simulink model "Simulation_1_3_dof"  (R2025a)
settings: Solver=VariableStepAuto  StartTime=0.0  StopTime=2000  FixedStep=1e-3  RelTol=1e-3
model workspace (MAT data in the model file):
  L1 = 0.29412
  L2 = 0.366795
  data_in = [0 0 0.1183997 0.1183997 0.1183997 0.03355169 0.03355169 0.3118325 0.3118325 0.3118325 0.3118325 0.6475105 ... (368 elements, 1x368)]
  data_in2 = [0 0 0 -1.210024 -1.210024 -1.210024 -1.304783 -1.304783 -1.304783 -1.673209 -1.673209 -1.673209 ... (368 elements, 1x368)]
  data_inYZ = [3.321716 3.321716 2.118667 2.118667 2.118667 2.649823 2.649823 2.756135 2.756135 2.756135 2.756135 2.832357 ... (368 elements, 1x368)]
  g = 9.81
  m1 = 1.7875
  m2 = 1.0285
  m3 = 0.3575
  m3_new = 2.3575
  m3_state_input = [0 0 0 0 0 0 0 0 0 0 0 0 0 0 0 0 0 0 0 0 0 0 0 0 0 0 0 0 0 0 0 0 0 0 0 0 0 0 0 0 0 0 0 0 0 0 0 0 0 0 0 0 0 0 0 0 0 0 0 0 0 0 0 0 0 0 0 0 0 0 0 0 0 0 0 0 0 0 0 0 0 0 0 0 0 0 0 0 0 0 0 0 0 0 0 0 0 0 0 0 0 0 0 0 0 0 0 0 0 0 0 0 0 0 0 0 0 0 0 0 0 0 0 0 0 0 0 0 0 0 0 0 0 0 0 0 0 0 0 0 0 0 0 0 0 0 0 0 0 0 0 0 0 0 0 0 0 0 0 0 0 0 0 0 0 0 0 0 0 0 0 0 0 0 0 0 0 0 0 0 0 0 0 0 0 0 0 0 0 0 0 0 0 0 0 0 0 0 0 0 0 0 0 0 0 0 0 0 0 0 0 0 0 0 0 0 0 0 0 0 0 0 0 0 0 0 0 0 0 0 0 0 0 0 0 0 0 0 0 0 0 0 0 0 0 0 0 0 0 0 0 0 0 0 0 0 0 0 0 0 0 0 0 0 0 0 0 0 0 0 0 0 0 0 0 0 0 0 0 0 0 0 0 0 0 0 0 0 0 0 0 0 0 0 0 0 0 0 0 0 0 0 0 0 0 0 0 0 0 0 0 0 0 0 0 0 0 0 0 0 0 0 0 0 0 0 0 0 0 0 0 0 0 0 0 0 0 0 0 0 0 0 0 0 0 0 0 0 0 0 0 0 0 0 0 0 0 0 0 0 0 0 0 0 0 0 0 0]
  trial_length = 12.6
libraries: simulink x1, slctrl_adaptive x1
settings Model: Creator=Queen  LastModifiedBy=jaanr
settings SolverCC: MaxConsecutiveMinStep=20  ZeroCrossAlgorithm=Adaptive
settings DataIOCC: SaveState=on
settings DebuggingCC: SignalInfNanChecking=warning  AlgebraicLoopMsg=none  IgnoredZcDiagnostic=none  SolverPrmCheckMsg=warning  CheckMatrixSingularityMsg=warning  StateNameClashWarn=warning  UnderSpecifiedDimensionMsg=warning

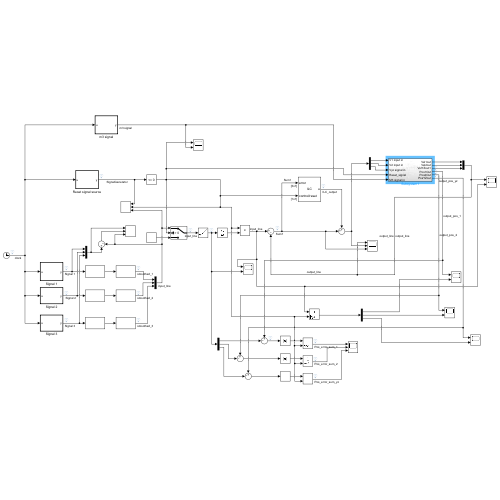
[thumbnail: Simulink's stored preview of the top-level diagram]
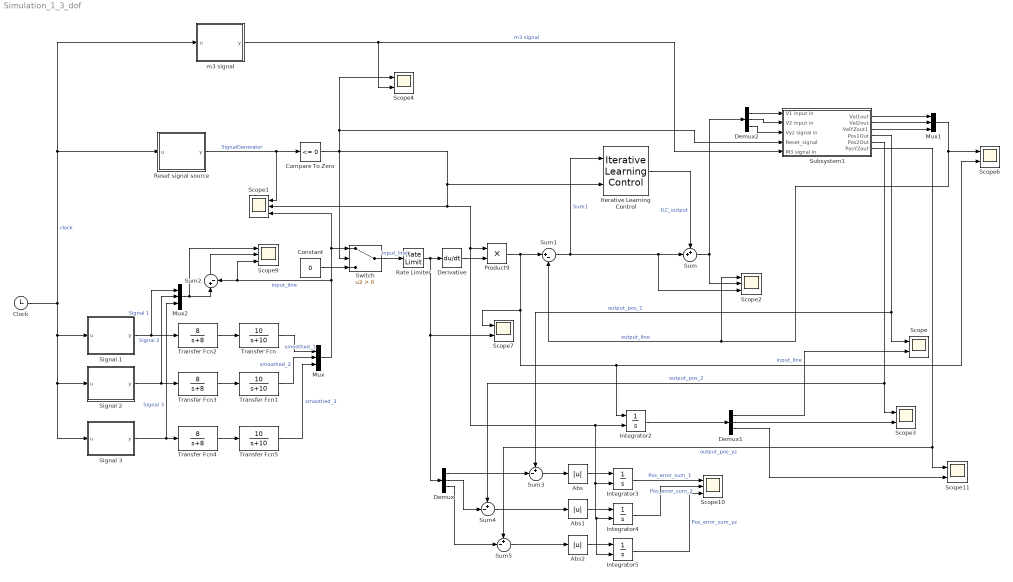
== system Simulation_1_3_dof ==
  Abs : Abs  SaturateOnIntegerOverflow=off
  Abs1 : Abs  SaturateOnIntegerOverflow=off
  Abs2 : Abs  SaturateOnIntegerOverflow=off
  Clock : Clock
  Compare To Zero : simulink/Logic and Bit Operations/Compare To Zero  relop=<=  OutDataTypeStr=boolean
  Constant : Constant  Value=0
  Demux : Demux  Outputs=3
  Demux1 : Demux  Outputs=3
  Demux2 : Demux  Outputs=3
  Derivative : Derivative
  Integrator{2..5} (4 alike) : Integrator  ExternalReset=either
  Iterative Learning Control : slctrl_adaptive/Iterative Learning Control  Ts=0.004  Tspan=trial_length  dataType=double  Algorithm=Model based ILC  gamma_p=1  gamma_d=0  ModelTimeDomain=Continuous time  A=[0 0 0; 0 0 0; 0 0 0]  B=[1 0 0; 0 1 0; 0 0 1]  C=[1 0 0; 0 1 0; 0 0 1]  ModelBasedILCType=Inverse-model based  gamma_inverse=1.9  gamma_grad=1  LPFEnable=on  tau=10
      settings: LibrarySourceBlock=slctrlblks/Adaptive Control/Iterative Learning Control
  Mux : Mux  Inputs=3
  Mux1 : Mux  Inputs=3
  Mux2 : Mux  Inputs=3
  Product9 : Product
  Rate Limiter : RateLimiter  RisingSlewLimit=100000  FallingSlewLimit=-100000  SampleTimeMode=inherited
  Reset signal source : MATLAB Function  StartFcn=const = data_in;  TreatAsAtomicUnit=on
  Scope{,3..4,6..7,11} (6 alike) : Scope  NumInputPorts=2
      Scope settings: ActiveDisplayYMinimum=-13.826115820369353  ActiveDisplayYMaximum=226.98217036515493
      Scope11 settings: ActiveDisplayYMinimum=-0.18701704840304334  ActiveDisplayYMaximum=1.1318992906932446  DataLoggingVariableName=ScopeData8
      Scope3 settings: ActiveDisplayYMinimum=-8.2804975413162367  ActiveDisplayYMaximum=200.54991353193529  DataLoggingVariableName=ScopeData3
      Scope4 settings: ActiveDisplayYMinimum=0.10884484415759765  ActiveDisplayYMaximum=4.3831313228801481
      Scope6 settings: ActiveDisplayYMinimum=-322.72558200957525  ActiveDisplayYMaximum=537.26898968089313  DataLoggingVariableName=ScopeData2
      Scope7 settings: ActiveDisplayYMinimum=-257.38444532138942  ActiveDisplayYMaximum=191.12119574725739  DataLoggingVariableName=ScopeData4
  Scope{1..2,9..10} (4 alike) : Scope  NumInputPorts=3
      Scope1 settings: ActiveDisplayYMinimum=80.127820191653512  ActiveDisplayYMaximum=87.873782524375827
      Scope10 settings: ActiveDisplayYMinimum=-1  ActiveDisplayYMaximum=1  DataLoggingVariableName=ScopeData7
      Scope2 settings: ActiveDisplayYMinimum=13.345255866197224  ActiveDisplayYMaximum=15.321548211532381  DataLoggingVariableName=ScopeData2
      Scope9 settings: ActiveDisplayYMinimum=-59.300205634382507  ActiveDisplayYMaximum=210.11663457106687  DataLoggingVariableName=ScopeData5
  Signal 1 : MATLAB Function  StartFcn=const = data_in;  TreatAsAtomicUnit=on
  Signal 2 : MATLAB Function  TreatAsAtomicUnit=on
  Signal 3 : MATLAB Function  TreatAsAtomicUnit=on
  Subsystem1 : Subsystem
  Sum : Sum  Inputs=++|
  Sum1 : Sum  Inputs=|+-
  Sum2 : Sum  Inputs=|+-
  Sum3 : Sum  Inputs=+-|
  Sum4 : Sum  Inputs=+-|
  Sum5 : Sum  Inputs=+-|
  Switch : Switch  Criteria=u2 > Threshold  SaturateOnIntegerOverflow=off  InputSameDT=off
  Transfer Fcn : TransferFcn  Numerator=[10]  Denominator=[1 10]
  Transfer Fcn1 : TransferFcn  Numerator=[10]  Denominator=[1 10]
  Transfer Fcn2 : TransferFcn  Numerator=[8]  Denominator=[1 8]
  Transfer Fcn3 : TransferFcn  Numerator=[8]  Denominator=[1 8]
  Transfer Fcn4 : TransferFcn  Numerator=[8]  Denominator=[1 8]
  Transfer Fcn5 : TransferFcn  Numerator=[10]  Denominator=[1 10]
  m3 signal : MATLAB Function  StartFcn=const = data_in;  TreatAsAtomicUnit=on
  wires:
  Constant/1 -> Switch/3
  Reset signal source/1(y) -> Scope1/1, Compare To Zero/1  "SignalGenerator"
  Compare To Zero/1 -> Integrator5/2, Integrator4/2, Integrator3/2, Integrator2/2, Product9/1, Scope1/2, Iterative Learning Control/2, Subsystem1/4(Reset_signal), Scope4/1, Switch/2
  Product9/1 -> Integrator2/1, Scope6/2, Scope7/1, Sum1/1  "input_line"
  Sum1/1 -> Sum/2, Scope2/3, Iterative Learning Control/1  "Sum1"
  Sum/1 -> Scope2/2, Demux2/1
  Mux1/1 -> Sum1/2, Scope2/1, Scope6/1  "output_line"
  Clock/1 -> m3 signal/1(u), Reset signal source/1(u), Signal 3/1(u), Signal 2/1(u), Signal 1/1(u)  "clock"
  Subsystem1/4(Pos1Out) -> Scope/1, Sum3/1  "output_pos_1"
  Subsystem1/5(Pos2Out) -> Sum4/1, Scope3/1  "output_pos_2"
  Demux1/1 -> Scope/2
  Demux1/2 -> Scope3/2
  Signal 2/1(y) -> Transfer Fcn3/1, Mux2/2  "Signal 2"
  Subsystem1/1(Vel1out) -> Mux1/1
  Subsystem1/2(Vel2out) -> Mux1/2
  Demux2/1 -> Subsystem1/1(V1 input in)
  Demux2/2 -> Subsystem1/2(V2 input in)
  Iterative Learning Control/1 -> Sum/1  "ILC_output"
  Integrator2/1 -> Demux1/1
  Switch/1 -> Rate Limiter/1  "input_line"
  Derivative/1 -> Product9/2
  Rate Limiter/1 -> Derivative/1, Demux/1, Scope7/2
  Signal 1/1(y) -> Transfer Fcn2/1, Mux2/1  "Signal 1"
  Mux/1 -> Scope9/3, Sum2/2, Scope1/3, Switch/1  "input_line"
  Transfer Fcn/1 -> Mux/1  "smoothed_1"
  Transfer Fcn1/1 -> Mux/2  "smoothed_2"
  Mux2/1 -> Sum2/1, Scope9/1
  Sum2/1 -> Scope9/2
  Transfer Fcn2/1 -> Transfer Fcn/1
  Transfer Fcn3/1 -> Transfer Fcn1/1
  m3 signal/1(y) -> Scope4/2, Subsystem1/5(M3 signal in)  "m3 signal"
  Demux/1 -> Sum3/2
  Demux/2 -> Sum4/2
  Sum3/1 -> Abs/1
  Sum4/1 -> Abs1/1
  Integrator3/1 -> Scope10/1  "Pos_error_sum_1"
  Integrator4/1 -> Scope10/2  "Pos_error_sum_2"
  Abs/1 -> Integrator3/1
  Abs1/1 -> Integrator4/1
  Signal 3/1(y) -> Transfer Fcn4/1, Mux2/3  "Signal 3"
  Transfer Fcn4/1 -> Transfer Fcn5/1
  Transfer Fcn5/1 -> Mux/3  "smoothed_3"
  Demux/3 -> Sum5/2
  Subsystem1/3(VelYZout1) -> Mux1/3
  Demux1/3 -> Scope11/2
  Subsystem1/6(PosYZout) -> Sum5/1, Scope11/1  "output_pos_yz"
  Sum5/1 -> Abs2/1
  Abs2/1 -> Integrator5/1
  Integrator5/1 -> Scope10/3  "Pos_error_sum_yz"
  Demux2/3 -> Subsystem1/3(Vyz signal in)

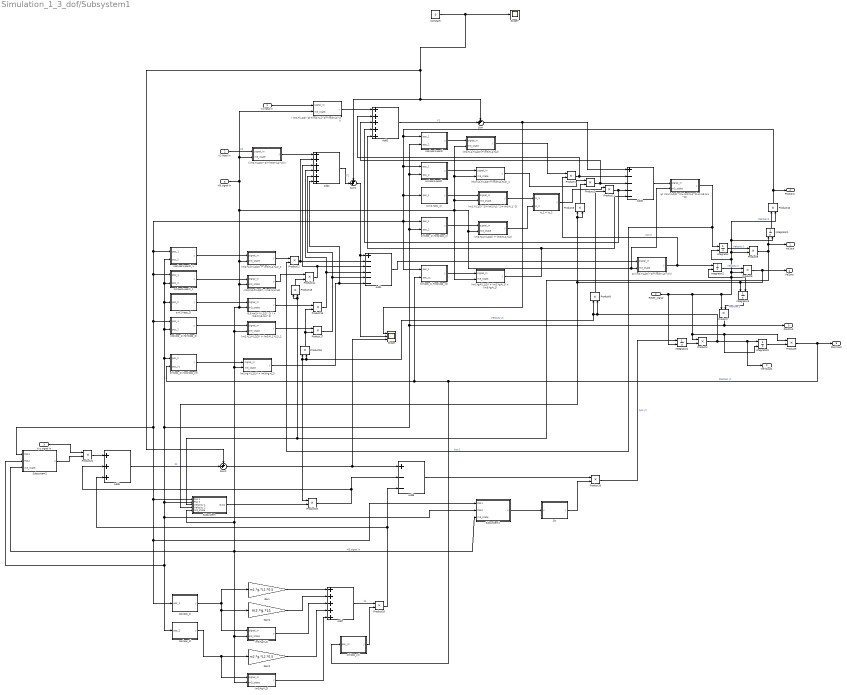
== system Simulation_1_3_dof/Subsystem1 ==
  V1 input in : Inport
  V2 input in : Inport  Port=2
  Vyz signal in : Inport  Port=3
  Reset_signal : Inport  Port=4
  M3 signal in : Inport  Port=5
  ( (m1.*(L1/2)^2)+(m2.*L1^2)+(m3.*L1^2)) : MATLAB Function  TreatAsAtomicUnit=on
  ((m2.*(L2/2)^2)+(m3.*(L2^2))) : MATLAB Function  TreatAsAtomicUnit=on
  (0.5.*m2.* ((L2/2)^2) ) + (0.5.*m3.*L2^2) : MATLAB Function  TreatAsAtomicUnit=on
  (m1.*(L1/2)^2)+(m2.*L1^2)+(m3.*L1^2) : MATLAB Function  TreatAsAtomicUnit=on
  (m1.*g.*(L1/2)) + (m2.*g.*L1) + (m3.*g.*L1) : MATLAB Function  TreatAsAtomicUnit=on
  (m2.*L1.*(L2/2)) + (m3.*L1.*L2) : MATLAB Function  TreatAsAtomicUnit=on
  (m2.*L1.*(L2/2)) + (m3.*L1.*L2)_1 : MATLAB Function  TreatAsAtomicUnit=on
  (m2.*L1.*(L2/2)) + (m3.*L1.*L2)_2 : MATLAB Function  TreatAsAtomicUnit=on
  (m2.*L1.*(L2/2))+(m3.*L1.*L2) : MATLAB Function  TreatAsAtomicUnit=on
  (m2.*L1.*(L2/2))+(m3.*L1.*L2)_1 : MATLAB Function  TreatAsAtomicUnit=on
  (m2.*g.*(L2/2)) + (m3.*g.*L2) : MATLAB Function  TreatAsAtomicUnit=on
  (m3.*g.*L1) : MATLAB Function  TreatAsAtomicUnit=on
  (m3.*g.*L2) : MATLAB Function  TreatAsAtomicUnit=on
  -(m2.*L1.*(L2/2)) - (m3.*L1.*L2) : MATLAB Function  TreatAsAtomicUnit=on
  1/( (m1.*(L1/2)^2)+(m2.*L1^2)+(m3.*L1^2)) : MATLAB Function  TreatAsAtomicUnit=on
  1/( (m2.*(L2/2)^2)+(m3.*(L2^2))) : MATLAB Function  TreatAsAtomicUnit=on
  1/u : MATLAB Function  TreatAsAtomicUnit=on
  Add1 : Sum  Inputs=+-----
  Add2 : Sum  Inputs=+++++
  Add3 : Sum  Inputs=+----
  Add4 : Sum  Inputs=++++++
  Add5 : Sum  Inputs=+++
  Add6 : Sum  Inputs=+--
  Add7 : Sum  Inputs=+++++
  Constant : Constant  Value=0
  Gain : Gain  Gain=m1.*g.*L1.*0.5
  Gain1 : Gain  Gain=m2.*g.*L1
  Gain2 : Gain  Gain=m2.*g.*L2.*0.5
  Integrator{,1..5} (6 alike) : Integrator  ExternalReset=either
  Product{1..21} (21 alike) : Product
  Scope : Scope  NumInputPorts=3
      settings: DataLoggingVariableName=ScopeData9
  Scope7 : Scope
      settings: ActiveDisplayYMinimum=-1  ActiveDisplayYMaximum=1  DataLoggingVariableName=ScopeData6
  Subsystem : Subsystem
  Subsystem1 : Subsystem
  Subsystem2 : Subsystem
  Sum : Sum  Inputs=++|
  Sum1 : Sum  Inputs=++|
  Sum2 : Sum  Inputs=++|
  cos(pos1-pos2) : MATLAB Function  TreatAsAtomicUnit=on
  cos(pos1-pos2)_1 : MATLAB Function  TreatAsAtomicUnit=on
  cos(pos_1) : MATLAB Function  TreatAsAtomicUnit=on
  cos(pos_1).*sin(pos_2) : MATLAB Function  TreatAsAtomicUnit=on
  cos(pos_2) : MATLAB Function  TreatAsAtomicUnit=on
  in_1 + in_2 : MATLAB Function  TreatAsAtomicUnit=on
  sin(2.*pos_1) : MATLAB Function  TreatAsAtomicUnit=on
  sin(2.*pos_2) : MATLAB Function  TreatAsAtomicUnit=on
  sin(pos1-pos2) : MATLAB Function  TreatAsAtomicUnit=on
  sin(pos1-pos2)_1 : MATLAB Function  TreatAsAtomicUnit=on
  sin(pos_1).*cos(pos_2) : MATLAB Function  TreatAsAtomicUnit=on
  sin(pos_1).*cos(pos_yz) : MATLAB Function  TreatAsAtomicUnit=on
  sin(pos_2).*cos(pos_yz) : MATLAB Function  TreatAsAtomicUnit=on
  sin(pos_yz) : MATLAB Function  TreatAsAtomicUnit=on
  Vel1out : Outport
  Vel2out : Outport  Port=2
  VelYZout1 : Outport  Port=3
  Pos1Out : Outport  Port=4
  Pos2Out : Outport  Port=5
  PosYZout : Outport  Port=6
  wires:
  Product9/1 -> Vel1out/1, Integrator1/1, Subsystem/3(Velocity 1), Product13/2, Product13/1
  Product6/1 -> Vel2out/1, Subsystem/4(Velocity 2), Product3/2, Product3/1, Integrator3/1
  Add3/1 -> 1/( (m1.*(L1/2)^2)+(m2.*L1^2)+(m3.*L1^2))/1(signal_in)
  1/( (m1.*(L1/2)^2)+(m2.*L1^2)+(m3.*L1^2))/1(y) -> Product12/2, Integrator/1  "Acc 1"
  Product10/1 -> cos(pos1-pos2)/1(pos_1), sin(pos1-pos2)/1(pos_1), sin(pos_1).*cos(pos_yz)/1(pos_1), cos(pos_1).*sin(pos_2)/1(pos_1), Subsystem1/1(Pos1), cos(pos_1)/1(pos_1), Subsystem/1(Pos 1), Subsystem2/1(Pos1), sin(pos1-pos2)_1/1(pos_1), cos(pos1-pos2)_1/1(pos_1), sin(pos_1).*cos(pos_2)/1(pos_1), sin(2.*pos_1)/1(pos_1), Pos1Out/1
  Product7/1 -> cos(pos_1).*sin(pos_2)/2(pos_2), sin(2.*pos_2)/1(pos_2), sin(pos1-pos2)_1/2(pos_2), cos(pos1-pos2)_1/2(pos_2), sin(pos_2).*cos(pos_yz)/1(pos_2), Subsystem2/2(Pos2), cos(pos_2)/1(pos_2), Subsystem1/2(Pos2), Subsystem/2(Pos 2), sin(pos1-pos2)/2(pos_2), cos(pos1-pos2)/2(pos_2), sin(pos_1).*cos(pos_2)/2(pos_2), Pos2Out/1
  1/( (m2.*(L2/2)^2)+(m3.*(L2^2)))/1(y) -> Product1/2, Integrator2/1  "Acc 2"
  Add1/1 -> 1/( (m2.*(L2/2)^2)+(m3.*(L2^2)))/1(signal_in)
  ( (m1.*(L1/2)^2)+(m2.*L1^2)+(m3.*L1^2))/1(y) -> Add2/1
  V1 input in/1 -> ( (m1.*(L1/2)^2)+(m2.*L1^2)+(m3.*L1^2))/1(signal_in)
  V2 input in/1 -> ((m2.*(L2/2)^2)+(m3.*(L2^2)))/1(signal_in)  "F2"
  ((m2.*(L2/2)^2)+(m3.*(L2^2)))/1(y) -> Add4/1
  Sum/1 -> Scope/1, Add3/1
  Constant/1 -> Sum2/1, Sum1/1, Sum/1, Scope7/1
  Sum1/1 -> Scope/2, Add1/1
  Add2/1 -> Sum/2  "F1"
  Add4/1 -> Sum1/2  "F2"
  Integrator/1 -> Product9/1  "Velocity 1"
  Integrator1/1 -> Product10/1  "Position 1"
  Integrator2/1 -> Product6/1  "Velocity 2"
  Integrator3/1 -> Product7/2  "Position 2"
  Reset_signal/1 -> Integrator4/2, Product10/2, Integrator1/2, Product9/2, Integrator/2, Product6/2, Integrator3/2, Integrator2/2, Product7/1, Product5/1, Integrator5/2, Product4/1
  M3 signal in/1 -> (m1.*g.*(L1/2)) + (m2.*g.*L1) + (m3.*g.*L1)/2(m3_state), 1/( (m1.*(L1/2)^2)+(m2.*L1^2)+(m3.*L1^2))/2(m3_state), 1/( (m2.*(L2/2)^2)+(m3.*(L2^2)))/2(m3_state), (m2.*L1.*(L2/2)) + (m3.*L1.*L2)/2(m3_state), (m1.*(L1/2)^2)+(m2.*L1^2)+(m3.*L1^2)/2(m3_state), (m2.*L1.*(L2/2))+(m3.*L1.*L2)/2(m3_state), (m2.*L1.*(L2/2))+(m3.*L1.*L2)_1/2(m3_state), -(m2.*L1.*(L2/2)) - (m3.*L1.*L2)/2(m3_state), (0.5.*m2.* ((L2/2)^2) ) + (0.5.*m3.*L2^2)/2(m3_state), (m2.*L1.*(L2/2)) + (m3.*L1.*L2)_2/2(m3_state), (m2.*g.*(L2/2)) + (m3.*g.*L2)/2(m3_state), Subsystem1/3(m3_state), (m3.*g.*L2)/2(m3_state), (m3.*g.*L1)/2(m3_state), Subsystem2/3(m3_state), Subsystem/5(m3_state), (m2.*L1.*(L2/2)) + (m3.*L1.*L2)_1/2(m3_state), ( (m1.*(L1/2)^2)+(m2.*L1^2)+(m3.*L1^2))/2(m3_state), ((m2.*(L2/2)^2)+(m3.*(L2^2)))/2(m3_state)  "M3 signal in"
  cos(pos1-pos2)/1(y) -> (m2.*L1.*(L2/2))+(m3.*L1.*L2)/1(signal_in)
  (m2.*L1.*(L2/2))+(m3.*L1.*L2)/1(y) -> Product1/1
  Product1/1 -> Add2/2, Add3/2
  sin(pos1-pos2)/1(y) -> (m2.*L1.*(L2/2))+(m3.*L1.*L2)_1/1(signal_in)
  (m2.*L1.*(L2/2))+(m3.*L1.*L2)_1/1(y) -> Product2/1
  Product3/1 -> Product2/2
  Product2/1 -> Add2/3, Add3/3
  sin(2.*pos_1)/1(y) -> (m1.*(L1/2)^2)+(m2.*L1^2)+(m3.*L1^2)/1(signal_in)
  (m1.*(L1/2)^2)+(m2.*L1^2)+(m3.*L1^2)/1(y) -> in_1 + in_2/1(in_1)
  sin(pos_1).*cos(pos_2)/1(y) -> (m2.*L1.*(L2/2)) + (m3.*L1.*L2)/1(signal_in)
  (m2.*L1.*(L2/2)) + (m3.*L1.*L2)/1(y) -> in_1 + in_2/2(in_2)
  Product20/1 -> Integrator4/1  "Acc yz"
  Integrator4/1 -> Product4/2
  Product4/1 -> VelYZout1/1, Integrator5/1, Product8/2, Product19/1, Product16/1, Product16/2, Product8/1  "Velocity yz"
  Integrator5/1 -> Product5/2
  Product5/1 -> PosYZout/1, sin(pos_yz)/1(pos_yz), sin(pos_1).*cos(pos_yz)/2(pos_yz), sin(pos_2).*cos(pos_yz)/2(pos_yz)  "Position yz"
  in_1 + in_2/1(y) -> Product11/1
  Product8/1 -> Product11/2
  Product11/1 -> Add2/4, Add3/4
  sin(pos_1).*cos(pos_yz)/1(y) -> (m1.*g.*(L1/2)) + (m2.*g.*L1) + (m3.*g.*L1)/1(signal_in)
  (m1.*g.*(L1/2)) + (m2.*g.*L1) + (m3.*g.*L1)/1(y) -> Add3/5, Add2/5
  cos(pos1-pos2)_1/1(y) -> (m2.*L1.*(L2/2)) + (m3.*L1.*L2)_1/1(signal_in)
  (m2.*L1.*(L2/2)) + (m3.*L1.*L2)_1/1(y) -> Product12/1
  Product12/1 -> Add1/2, Add4/2
  sin(pos1-pos2)_1/1(y) -> -(m2.*L1.*(L2/2)) - (m3.*L1.*L2)/1(signal_in)
  -(m2.*L1.*(L2/2)) - (m3.*L1.*L2)/1(y) -> Product14/1
  Product13/1 -> Product14/2
  Product14/1 -> Add1/3, Add4/3
  sin(2.*pos_2)/1(y) -> (0.5.*m2.* ((L2/2)^2) ) + (0.5.*m3.*L2^2)/1(signal_in)
  (0.5.*m2.* ((L2/2)^2) ) + (0.5.*m3.*L2^2)/1(y) -> Product15/1
  Product15/1 -> Add4/4, Add1/4
  cos(pos_1).*sin(pos_2)/1(y) -> (m2.*L1.*(L2/2)) + (m3.*L1.*L2)_2/1(signal_in)
  (m2.*L1.*(L2/2)) + (m3.*L1.*L2)_2/1(y) -> Product17/1
  Product16/1 -> Product15/2, Product17/2
  Product17/1 -> Add4/5, Add1/5
  sin(pos_2).*cos(pos_yz)/1(y) -> (m2.*g.*(L2/2)) + (m3.*g.*L2)/1(signal_in)
  (m2.*g.*(L2/2)) + (m3.*g.*L2)/1(y) -> Add4/6, Add1/6
  Add5/1 -> Sum2/2  "F1"
  Sum2/1 -> Scope/3, Add6/1
  cos(pos_1)/1(y) -> (m3.*g.*L1)/1(signal_in), Gain1/1, Gain/1
  cos(pos_2)/1(y) -> (m3.*g.*L2)/1(signal_in), Gain2/1
  Gain/1 -> Add7/1
  Gain1/1 -> Add7/2
  (m3.*g.*L1)/1(y) -> Add7/3
  Gain2/1 -> Add7/4
  (m3.*g.*L2)/1(y) -> Add7/5
  Add7/1 -> Product18/1  "F1"
  sin(pos_yz)/1(y) -> Product18/2
  Product18/1 -> Add5/3, Add6/3
  Subsystem/1(Out1) -> Product19/2
  Product19/1 -> Add6/2, Add5/2
  Subsystem1/1(u) -> 1/u/1(u)
  Add6/1 -> Product20/1
  1/u/1(y) -> Product20/2
  Subsystem2/1(u) -> Product21/2
  Vyz signal in/1 -> Product21/1
  Product21/1 -> Add5/1

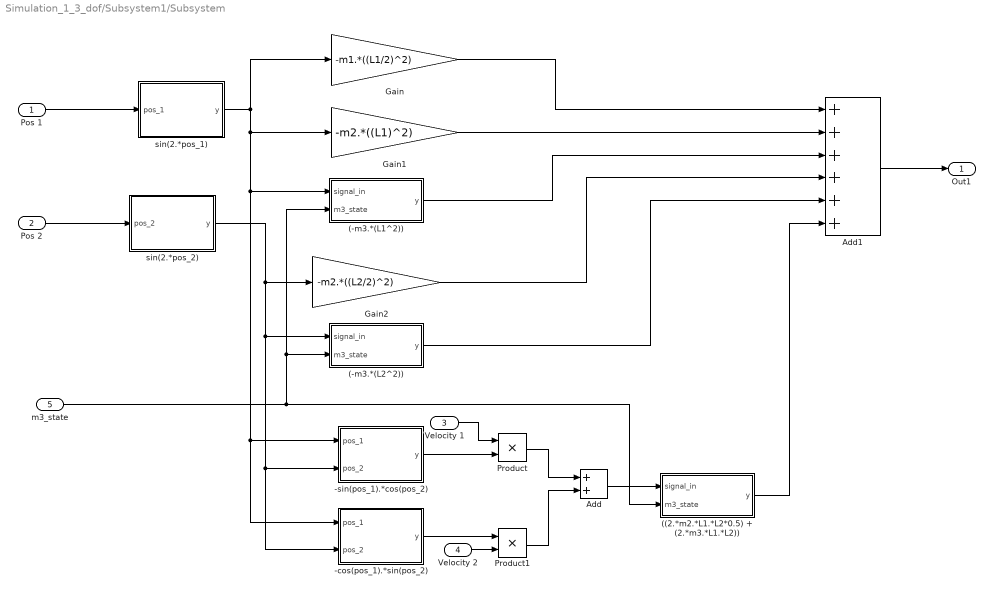
== system Simulation_1_3_dof/Subsystem1/Subsystem ==
  Pos 1 : Inport
  Pos 2 : Inport  Port=2
  Velocity 1 : Inport  Port=3
  Velocity 2 : Inport  Port=4
  m3_state : Inport  Port=5
  ((2.*m2.*L1.*L2*0.5) + (2.*m3.*L1.*L2)) : MATLAB Function  TreatAsAtomicUnit=on
  (-m3.*(L1^2)) : MATLAB Function  TreatAsAtomicUnit=on
  (-m3.*(L2^2)) : MATLAB Function  TreatAsAtomicUnit=on
  -cos(pos_1).*sin(pos_2) : MATLAB Function  TreatAsAtomicUnit=on
  -sin(pos_1).*cos(pos_2) : MATLAB Function  TreatAsAtomicUnit=on
  Add : Sum
  Add1 : Sum  Inputs=++++++
  Gain : Gain  Gain=-m1.*((L1/2)^2)
  Gain1 : Gain  Gain=-m2.*((L1)^2)
  Gain2 : Gain  Gain=-m2.*((L2/2)^2)
  Product : Product
  Product1 : Product
  sin(2.*pos_1) : MATLAB Function  TreatAsAtomicUnit=on
  sin(2.*pos_2) : MATLAB Function  TreatAsAtomicUnit=on
  Out1 : Outport
  wires:
  Pos 1/1 -> sin(2.*pos_1)/1(pos_1)
  sin(2.*pos_1)/1(y) -> Gain/1, (-m3.*(L1^2))/1(signal_in), -sin(pos_1).*cos(pos_2)/1(pos_1), -cos(pos_1).*sin(pos_2)/1(pos_1), Gain1/1
  m3_state/1 -> (-m3.*(L1^2))/2(m3_state), (-m3.*(L2^2))/2(m3_state), ((2.*m2.*L1.*L2*0.5) + (2.*m3.*L1.*L2))/2(m3_state)
  Pos 2/1 -> sin(2.*pos_2)/1(pos_2)
  sin(2.*pos_2)/1(y) -> -sin(pos_1).*cos(pos_2)/2(pos_2), -cos(pos_1).*sin(pos_2)/2(pos_2), (-m3.*(L2^2))/1(signal_in), Gain2/1
  -sin(pos_1).*cos(pos_2)/1(y) -> Product/2
  Velocity 1/1 -> Product/1
  Velocity 2/1 -> Product1/2
  -cos(pos_1).*sin(pos_2)/1(y) -> Product1/1
  Product/1 -> Add/1
  Product1/1 -> Add/2
  Add/1 -> ((2.*m2.*L1.*L2*0.5) + (2.*m3.*L1.*L2))/1(signal_in)
  Gain/1 -> Add1/1
  Gain1/1 -> Add1/2
  (-m3.*(L1^2))/1(y) -> Add1/3
  Gain2/1 -> Add1/4
  (-m3.*(L2^2))/1(y) -> Add1/5
  ((2.*m2.*L1.*L2*0.5) + (2.*m3.*L1.*L2))/1(y) -> Add1/6
  Add1/1 -> Out1/1

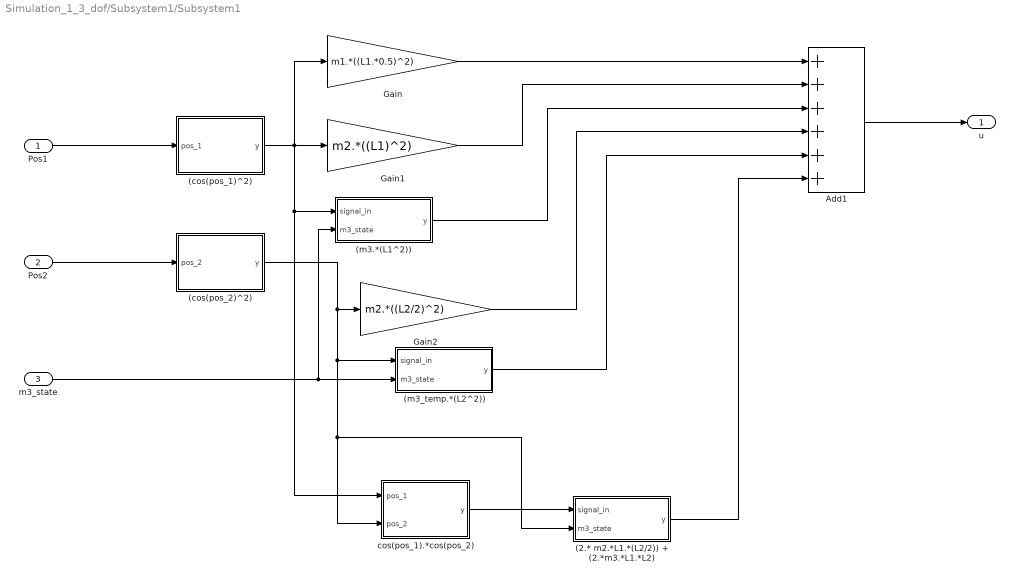
== system Simulation_1_3_dof/Subsystem1/Subsystem1 ==
  Pos1 : Inport
  Pos2 : Inport  Port=2
  m3_state : Inport  Port=3
  (2.* m2.*L1.*(L2/2)) + (2.*m3.*L1.*L2) : MATLAB Function  TreatAsAtomicUnit=on
  (cos(pos_1)^2) : MATLAB Function  TreatAsAtomicUnit=on
  (cos(pos_2)^2) : MATLAB Function  TreatAsAtomicUnit=on
  (m3.*(L1^2)) : MATLAB Function  TreatAsAtomicUnit=on
  (m3_temp.*(L2^2)) : MATLAB Function  TreatAsAtomicUnit=on
  Add1 : Sum  Inputs=++++++
  Gain : Gain  Gain=m1.*((L1.*0.5)^2)
  Gain1 : Gain  Gain=m2.*((L1)^2)
  Gain2 : Gain  Gain=m2.*((L2/2)^2)
  cos(pos_1).*cos(pos_2) : MATLAB Function  TreatAsAtomicUnit=on
  u : Outport
  wires:
  Pos1/1 -> (cos(pos_1)^2)/1(pos_1)
  (cos(pos_1)^2)/1(y) -> cos(pos_1).*cos(pos_2)/1(pos_1), (m3.*(L1^2))/1(signal_in), Gain1/1, Gain/1
  m3_state/1 -> (m3.*(L1^2))/2(m3_state), (m3_temp.*(L2^2))/2(m3_state)
  Pos2/1 -> (cos(pos_2)^2)/1(pos_2)
  (cos(pos_2)^2)/1(y) -> (2.* m2.*L1.*(L2/2)) + (2.*m3.*L1.*L2)/2(m3_state), cos(pos_1).*cos(pos_2)/2(pos_2), (m3_temp.*(L2^2))/1(signal_in), Gain2/1
  cos(pos_1).*cos(pos_2)/1(y) -> (2.* m2.*L1.*(L2/2)) + (2.*m3.*L1.*L2)/1(signal_in)
  Gain/1 -> Add1/1
  Gain1/1 -> Add1/2
  (m3.*(L1^2))/1(y) -> Add1/3
  Gain2/1 -> Add1/4
  (2.* m2.*L1.*(L2/2)) + (2.*m3.*L1.*L2)/1(y) -> Add1/6
  Add1/1 -> u/1
  (m3_temp.*(L2^2))/1(y) -> Add1/5

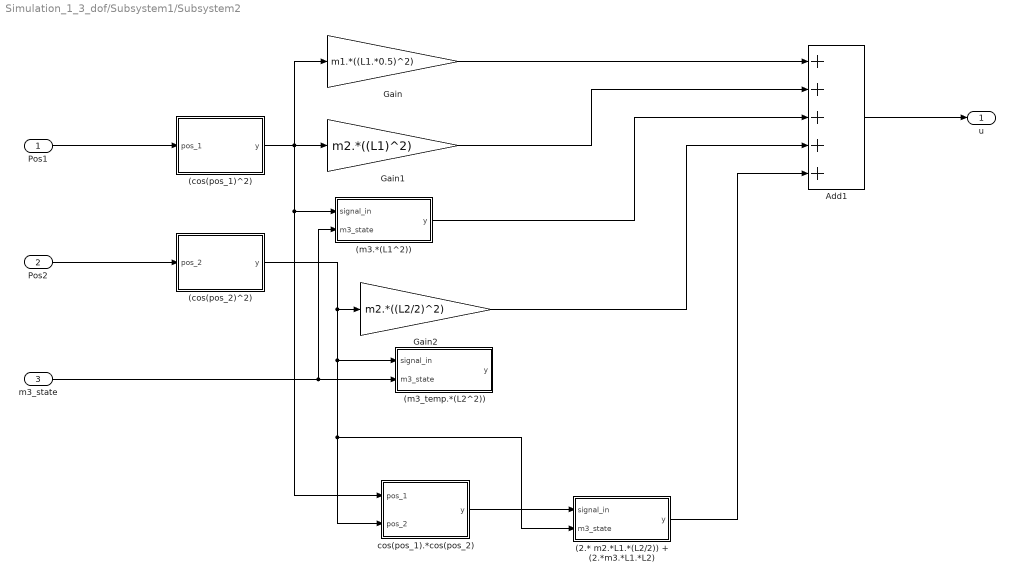
== system Simulation_1_3_dof/Subsystem1/Subsystem2 ==
  Pos1 : Inport
  Pos2 : Inport  Port=2
  m3_state : Inport  Port=3
  (2.* m2.*L1.*(L2/2)) + (2.*m3.*L1.*L2) : MATLAB Function  TreatAsAtomicUnit=on
  (cos(pos_1)^2) : MATLAB Function  TreatAsAtomicUnit=on
  (cos(pos_2)^2) : MATLAB Function  TreatAsAtomicUnit=on
  (m3.*(L1^2)) : MATLAB Function  TreatAsAtomicUnit=on
  (m3_temp.*(L2^2)) : MATLAB Function  TreatAsAtomicUnit=on
  Add1 : Sum  Inputs=+++++
  Gain : Gain  Gain=m1.*((L1.*0.5)^2)
  Gain1 : Gain  Gain=m2.*((L1)^2)
  Gain2 : Gain  Gain=m2.*((L2/2)^2)
  cos(pos_1).*cos(pos_2) : MATLAB Function  TreatAsAtomicUnit=on
  u : Outport
  wires:
  Pos1/1 -> (cos(pos_1)^2)/1(pos_1)
  (cos(pos_1)^2)/1(y) -> cos(pos_1).*cos(pos_2)/1(pos_1), (m3.*(L1^2))/1(signal_in), Gain1/1, Gain/1
  m3_state/1 -> (m3.*(L1^2))/2(m3_state), (m3_temp.*(L2^2))/2(m3_state)
  Pos2/1 -> (cos(pos_2)^2)/1(pos_2)
  (cos(pos_2)^2)/1(y) -> (2.* m2.*L1.*(L2/2)) + (2.*m3.*L1.*L2)/2(m3_state), cos(pos_1).*cos(pos_2)/2(pos_2), (m3_temp.*(L2^2))/1(signal_in), Gain2/1
  cos(pos_1).*cos(pos_2)/1(y) -> (2.* m2.*L1.*(L2/2)) + (2.*m3.*L1.*L2)/1(signal_in)
  Gain/1 -> Add1/1
  Gain1/1 -> Add1/2
  (m3.*(L1^2))/1(y) -> Add1/3
  Gain2/1 -> Add1/4
  (2.* m2.*L1.*(L2/2)) + (2.*m3.*L1.*L2)/1(y) -> Add1/5
  Add1/1 -> u/1

== matlab function Simulation_1_3_dof/Subsystem1/cos(pos1-pos2) ==
  data: y output; pos_1 input; pos_2 input
function y = fcn(pos_1, pos_2)

y = cos(pos_1-pos_2);

== matlab function Simulation_1_3_dof/Subsystem1/(m2.*L1.*(L2//2))+(m3.*L1.*L2) ==
  data: signal_in input; y output; m3_state input; m3 parameter; m3_new parameter; L1 parameter; m2 parameter; L2 parameter
function y  = fcn(signal_in,m3_state,m3, m3_new, L1, m2, L2)

m3_temp = 0;

if m3_state == 1
    m3_temp = m3_new;
else
    m3_temp = m3;
end

y = signal_in .* ((m2.*L1.*(L2/2))+(m3_temp.*L1.*L2));

== matlab function Simulation_1_3_dof/Subsystem1/sin(pos1-pos2) ==
  data: y output; pos_1 input; pos_2 input
function y = fcn(pos_1, pos_2)

y = sin(pos_1-pos_2);

== matlab function Simulation_1_3_dof/Subsystem1/(m2.*L1.*(L2//2))+(m3.*L1.*L2)_1 ==
  data: signal_in input; y output; m3_state input; m3 parameter; m3_new parameter; L1 parameter; m2 parameter; L2 parameter
function y  = fcn(signal_in,m3_state,m3, m3_new, L1, m2, L2)

m3_temp = 0;

if m3_state == 1
    m3_temp = m3_new;
else
    m3_temp = m3;
end

y = signal_in .* ((m2.*L1.*(L2/2))+(m3_temp.*L1.*L2));

== matlab function Simulation_1_3_dof/Subsystem1/sin(2.*pos_1) ==
  data: y output; pos_1 input
function y = fcn(pos_1)

y = sin(2.*pos_1);

== matlab function Simulation_1_3_dof/Subsystem1/(m1.*(L1//2)^2)+(m2.*L1^2)+(m3.*L1^2) ==
  data: signal_in input; y output; m3_state input; m3 parameter; m3_new parameter; L1 parameter; m2 parameter; m1 parameter
function y  = fcn(signal_in,m3_state,m3, m3_new, L1, m2, m1)

m3_temp = 0;

if m3_state == 1
    m3_temp = m3_new;
else
    m3_temp = m3;
end

y = signal_in .* ( (0.5.*m1.*(L1/2)^2) + (0.5.*m2.*L1^2) + (0.5.*m3_temp.*L1^2) );

== matlab function Simulation_1_3_dof/Subsystem1/in_1 + in_2 ==
  data: y output; in_1 input; in_2 input
function y = fcn(in_1, in_2)

y = in_1 + in_2;

== matlab function Simulation_1_3_dof/Subsystem1/sin(pos_1).*cos(pos_2) ==
  data: y output; pos_1 input; pos_2 input
function y = fcn(pos_1, pos_2)

y = sin(pos_1).*cos(pos_2);

== matlab function Simulation_1_3_dof/Subsystem1/(m2.*L1.*(L2//2)) + (m3.*L1.*L2) ==
  data: signal_in input; y output; m3_state input; m3 parameter; m3_new parameter; L1 parameter; m2 parameter; L2 parameter
function y  = fcn(signal_in,m3_state,m3, m3_new, L1, m2, L2)

m3_temp = 0;

if m3_state == 1
    m3_temp = m3_new;
else
    m3_temp = m3;
end

y = signal_in .* ( (m2.*L1.*(L2/2)) + (m3_temp.*L1.*L2) );

== matlab function Simulation_1_3_dof/Subsystem1/sin(pos_1).*cos(pos_yz) ==
  data: y output; pos_1 input; pos_yz input
function y = fcn(pos_1, pos_yz)

y = sin(pos_1).*cos(pos_yz);

== matlab function Simulation_1_3_dof/Signal 1 ==
  data: u input; y output; data_in parameter; trial_length parameter
function y = fcn(u, data_in, trial_length)

%u is the clock time input
x = mod(u, (trial_length+3));

%check_data = 0:0.01:10;
check_data = data_in;


y_temp = 0;

[numRows,numCols] = size(check_data);
loop = 1;

%disp(class(round((x./(step/2)).*numCols)))
i=round((x./(trial_length)).*numCols);
if i == 0
    i = 1;
end
if i>numCols
    i = numCols;
end
y_temp = check_data(1,i);



if x>=trial_length
    y = 0;
else
    y = y_temp;

end

== matlab function Simulation_1_3_dof/Subsystem1/(m1.*g.*(L1//2)) + (m2.*g.*L1) + (m3.*g.*L1) ==
  data: signal_in input; y output; m3_state input; m3 parameter; m3_new parameter; L1 parameter; m2 parameter; m1 parameter; g parameter
function y  = fcn(signal_in,m3_state,m3, m3_new, L1, m2, m1, g)

m3_temp = 0;

if m3_state == 1
    m3_temp = m3_new;
else
    m3_temp = m3;
end

y = signal_in .* ( (m1.*g.*(L1/2)) + (m2.*g.*L1) + (m3_temp.*g.*L1) );

== matlab function Simulation_1_3_dof/Subsystem1/cos(pos1-pos2)_1 ==
  data: y output; pos_1 input; pos_2 input
function y = fcn(pos_1, pos_2)

y = cos(pos_1-pos_2);

== matlab function Simulation_1_3_dof/Subsystem1/(m2.*L1.*(L2//2)) + (m3.*L1.*L2)_1 ==
  data: signal_in input; y output; m3_state input; m3 parameter; m3_new parameter; L1 parameter; m2 parameter; L2 parameter
function y  = fcn(signal_in,m3_state,m3, m3_new, L1, m2, L2)

m3_temp = 0;

if m3_state == 1
    m3_temp = m3_new;
else
    m3_temp = m3;
end

y = signal_in .* ( (m2.*L1.*(L2/2)) + (m3_temp.*L1.*L2) );

== matlab function Simulation_1_3_dof/Subsystem1/-(m2.*L1.*(L2//2)) - (m3.*L1.*L2) ==
  data: signal_in input; y output; m3_state input; m3 parameter; m3_new parameter; L1 parameter; m2 parameter; L2 parameter
function y  = fcn(signal_in,m3_state,m3, m3_new, L1, m2, L2)

m3_temp = 0;

if m3_state == 1
    m3_temp = m3_new;
else
    m3_temp = m3;
end

y = signal_in .* ( -(m2.*L1.*(L2/2)) - (m3_temp.*L1.*L2) );

== matlab function Simulation_1_3_dof/Subsystem1/sin(pos1-pos2)_1 ==
  data: y output; pos_1 input; pos_2 input
function y = fcn(pos_1, pos_2)

y = sin(pos_1-pos_2);

== matlab function Simulation_1_3_dof/Subsystem1/sin(2.*pos_2) ==
  data: y output; pos_2 input
function y = fcn(pos_2)

y = sin(2.*pos_2);

== matlab function Simulation_1_3_dof/Subsystem1/(0.5.*m2.* ((L2//2)^2) ) + (0.5.*m3.*L2^2) ==
  data: signal_in input; y output; m3_state input; m3 parameter; m3_new parameter; m2 parameter; L2 parameter
function y  = fcn(signal_in,m3_state,m3, m3_new, m2, L2)

m3_temp = 0;

if m3_state == 1
    m3_temp = m3_new;
else
    m3_temp = m3;
end

y = signal_in .* ( (0.5.*m2.* ((L2/2)^2) ) + (0.5.*m3_temp.*L2^2) );

== matlab function Simulation_1_3_dof/Subsystem1/cos(pos_1).*sin(pos_2) ==
  data: y output; pos_1 input; pos_2 input
function y = fcn(pos_1, pos_2)

y = cos(pos_1).*sin(pos_2);

== matlab function Simulation_1_3_dof/Subsystem1/(m2.*L1.*(L2//2)) + (m3.*L1.*L2)_2 ==
  data: signal_in input; y output; m3_state input; m3 parameter; m3_new parameter; L1 parameter; m2 parameter; L2 parameter
function y  = fcn(signal_in,m3_state,m3, m3_new, L1, m2, L2)

m3_temp = 0;

if m3_state == 1
    m3_temp = m3_new;
else
    m3_temp = m3;
end

y = signal_in .* ( (m2.*L1.*(L2/2)) + (m3_temp.*L1.*L2) );

== matlab function Simulation_1_3_dof/Signal 2 ==
  data: u input; y output; data_in2 parameter; trial_length parameter
function y = fcn(u, data_in2, trial_length)

%u is the clock time input

%u is the clock time input
x = mod(u, (trial_length+3));


%check_data = 0:0.01:10;
check_data = data_in2;


y_temp = 0;

[numRows,numCols] = size(check_data);
loop = 1;

%disp(class(round((x./(step/2)).*numCols)))
i=round((x./(trial_length)).*numCols);
if i == 0
    i = 1;
end
if i>numCols
    i = numCols;
end
y_temp = check_data(1,i);


if x>=trial_length
    y = 0;
else
    y = y_temp;

end

== matlab function Simulation_1_3_dof/Subsystem1/sin(pos_2).*cos(pos_yz) ==
  data: pos_2 input; y output; pos_yz input
function y = fcn(pos_2, pos_yz)

y = sin(pos_2).*cos(pos_yz);

== matlab function Simulation_1_3_dof/Subsystem1/(m2.*g.*(L2//2)) + (m3.*g.*L2) ==
  data: signal_in input; y output; m3_state input; m3 parameter; m3_new parameter; m2 parameter; L2 parameter; g parameter
function y  = fcn(signal_in,m3_state,m3, m3_new, m2, L2, g)

m3_temp = 0;

if m3_state == 1
    m3_temp = m3_new;
else
    m3_temp = m3;
end

y = signal_in .* ( (m2.*g.*(L2/2)) + (m3_temp.*g.*L2) );

== matlab function Simulation_1_3_dof/Subsystem1/cos(pos_1) ==
  data: y output; pos_1 input
function y = fcn(pos_1)

y = cos(pos_1);

== matlab function Simulation_1_3_dof/Subsystem1/cos(pos_2) ==
  data: y output; pos_2 input
function y = fcn(pos_2)

y = cos(pos_2);

== matlab function Simulation_1_3_dof/Subsystem1/(m3.*g.*L1) ==
  data: signal_in input; y output; m3_state input; m3 parameter; m3_new parameter; L1 parameter; g parameter
function y  = fcn(signal_in,m3_state,m3, m3_new, L1, g)

m3_temp = 0;

if m3_state == 1
    m3_temp = m3_new;
else
    m3_temp = m3;
end

y = signal_in .* (m3_temp.*g.*L1) ;

== matlab function Simulation_1_3_dof/Subsystem1/(m3.*g.*L2) ==
  data: signal_in input; y output; m3_state input; m3 parameter; m3_new parameter; L2 parameter; g parameter
function y  = fcn(signal_in,m3_state,m3, m3_new, L2, g)

m3_temp = 0;

if m3_state == 1
    m3_temp = m3_new;
else
    m3_temp = m3;
end

y = signal_in .* (m3_temp.*g.*L2) ;

== matlab function Simulation_1_3_dof/Subsystem1/sin(pos_yz) ==
  data: y output; pos_yz input
function y = fcn(pos_yz)


y = sin(pos_yz);

== matlab function Simulation_1_3_dof/Subsystem1/Subsystem/sin(2.*pos_1) ==
  data: y output; pos_1 input
function y = fcn(pos_1)

y = sin(2.*pos_1);

== matlab function Simulation_1_3_dof/Subsystem1/Subsystem/(-m3.*(L1^2)) ==
  data: signal_in input; y output; m3_state input; m3 parameter; m3_new parameter; L1 parameter
function y  = fcn(signal_in,m3_state,m3, m3_new, L1)

m3_temp = 0;

if m3_state == 1
    m3_temp = m3_new;
else
    m3_temp = m3;
end

y = signal_in .* (-m3_temp.*(L1^2)) ;

== matlab function Simulation_1_3_dof/Reset signal source ==
  data: u input; y output; trial_length parameter
function y = fcn(u, trial_length)

%u is the clock time input
x = mod(u, (trial_length+3));


if x>=trial_length
    y = 1;
else
    y = -1;

end

== matlab function Simulation_1_3_dof/Subsystem1/Subsystem/sin(2.*pos_2) ==
  data: y output; pos_2 input
function y = fcn(pos_2)

y = sin(2.*pos_2);

== matlab function Simulation_1_3_dof/Subsystem1/Subsystem/(-m3.*(L2^2)) ==
  data: signal_in input; y output; m3_state input; m3 parameter; m3_new parameter; L2 parameter
function y  = fcn(signal_in,m3_state,m3, m3_new, L2)

m3_temp = 0;

if m3_state == 1
    m3_temp = m3_new;
else
    m3_temp = m3;
end

y = signal_in .* (-m3_temp.*(L2^2)) ;

== matlab function Simulation_1_3_dof/Subsystem1/Subsystem/-sin(pos_1).*cos(pos_2) ==
  data: y output; pos_1 input; pos_2 input
function y = fcn(pos_1, pos_2)

y = -sin(pos_1).*cos(pos_2);

== matlab function Simulation_1_3_dof/Subsystem1/Subsystem/-cos(pos_1).*sin(pos_2) ==
  data: y output; pos_1 input; pos_2 input
function y = fcn(pos_1, pos_2)

y = -cos(pos_1).*sin(pos_2);

== matlab function Simulation_1_3_dof/Subsystem1/Subsystem/((2.*m2.*L1.*L2*0.5) + (2.*m3.*L1.*L2)) ==
  data: signal_in input; y output; m3_state input; m3 parameter; m3_new parameter; L2 parameter; m2 parameter; L1 parameter
function y  = fcn(signal_in,m3_state,m3, m3_new, L2, m2, L1)

m3_temp = 0;

if m3_state == 1
    m3_temp = m3_new;
else
    m3_temp = m3;
end

y = signal_in .* ((2.*m2.*L1.*L2*0.5) + (2.*m3_temp.*L1.*L2)) ;

== matlab function Simulation_1_3_dof/Subsystem1/Subsystem1/(cos(pos_1)^2) ==
  data: y output; pos_1 input
function y = fcn(pos_1)

y = (cos(pos_1)^2);

== matlab function Simulation_1_3_dof/Subsystem1/Subsystem1/(cos(pos_2)^2) ==
  data: y output; pos_2 input
function y = fcn(pos_2)

y = (cos(pos_2)^2);

== matlab function Simulation_1_3_dof/Subsystem1/Subsystem1/(m3.*(L1^2)) ==
  data: signal_in input; y output; m3_state input; m3 parameter; m3_new parameter; L1 parameter
function y  = fcn(signal_in,m3_state,m3, m3_new, L1)

m3_temp = 0;

if m3_state == 1
    m3_temp = m3_new;
else
    m3_temp = m3;
end

y = signal_in .* (m3_temp.*(L1^2)) ;

== matlab function Simulation_1_3_dof/Subsystem1/Subsystem1/(m3_temp.*(L2^2)) ==
  data: signal_in input; y output; m3_state input; m3 parameter; m3_new parameter; L2 parameter
function y  = fcn(signal_in,m3_state,m3, m3_new, L2)

m3_temp = 0;

if m3_state == 1
    m3_temp = m3_new;
else
    m3_temp = m3;
end

y = signal_in .* (m3_temp.*(L2^2)) ;

== matlab function Simulation_1_3_dof/Subsystem1/( (m1.*(L1//2)^2)+(m2.*L1^2)+(m3.*L1^2)) ==
  data: signal_in input; y output; m3_state input; m3 parameter; m3_new parameter; L1 parameter; m2 parameter; m1 parameter
function y  = fcn(signal_in,m3_state,m3, m3_new, L1, m2, m1)

m3_temp = 0;

if m3_state == 1
    m3_temp = m3_new;
else
    m3_temp = m3;
end

y = signal_in .* ((m1.*(L1/2)^2)+(m2.*L1^2)+(m3_temp.*L1^2));

== matlab function Simulation_1_3_dof/Subsystem1/Subsystem1/cos(pos_1).*cos(pos_2) ==
  data: y output; pos_1 input; pos_2 input
function y = fcn(pos_1, pos_2)

y = cos(pos_1).*cos(pos_2);

== matlab function Simulation_1_3_dof/Subsystem1/Subsystem1/(2.* m2.*L1.*(L2//2)) + (2.*m3.*L1.*L2) ==
  data: signal_in input; y output; m3_state input; m3 parameter; m3_new parameter; L1 parameter; m2 parameter; L2 parameter
function y  = fcn(signal_in,m3_state,m3, m3_new, L1, m2, L2)

m3_temp = 0;

if m3_state == 1
    m3_temp = m3_new;
else
    m3_temp = m3;
end

y = signal_in .* ( (2.* m2.*L1.*(L2/2)) + (2.*m3_temp.*L1.*L2) );

== matlab function Simulation_1_3_dof/Subsystem1/1//u ==
  data: y output; u input
function y = fcn(u)

y = 1/u;

== matlab function Simulation_1_3_dof/Subsystem1/Subsystem2/(2.* m2.*L1.*(L2//2)) + (2.*m3.*L1.*L2) ==
  data: signal_in input; y output; m3_state input; m3 parameter; m3_new parameter; L1 parameter; m2 parameter; L2 parameter
function y  = fcn(signal_in,m3_state,m3, m3_new, L1, m2, L2)

m3_temp = 0;

if m3_state == 1
    m3_temp = m3_new;
else
    m3_temp = m3;
end

y = signal_in .* ( (2.* m2.*L1.*(L2/2)) + (2.*m3_temp.*L1.*L2) );

== matlab function Simulation_1_3_dof/Subsystem1/Subsystem2/(cos(pos_1)^2) ==
  data: y output; pos_1 input
function y = fcn(pos_1)

y = (cos(pos_1)^2);

== matlab function Simulation_1_3_dof/Subsystem1/Subsystem2/(cos(pos_2)^2) ==
  data: y output; pos_2 input
function y = fcn(pos_2)

y = (cos(pos_2)^2);

== matlab function Simulation_1_3_dof/Subsystem1/Subsystem2/(m3.*(L1^2)) ==
  data: signal_in input; y output; m3_state input; m3 parameter; m3_new parameter; L1 parameter
function y  = fcn(signal_in,m3_state,m3, m3_new, L1)

m3_temp = 0;

if m3_state == 1
    m3_temp = m3_new;
else
    m3_temp = m3;
end

y = signal_in .* (m3_temp.*(L1^2)) ;

== matlab function Simulation_1_3_dof/Subsystem1/Subsystem2/(m3_temp.*(L2^2)) ==
  data: signal_in input; y output; m3_state input; m3 parameter; m3_new parameter; L2 parameter
function y  = fcn(signal_in,m3_state,m3, m3_new, L2)

m3_temp = 0;

if m3_state == 1
    m3_temp = m3_new;
else
    m3_temp = m3;
end

y = signal_in .* (m3_temp.*(L2^2)) ;

== matlab function Simulation_1_3_dof/Subsystem1/Subsystem2/cos(pos_1).*cos(pos_2) ==
  data: y output; pos_1 input; pos_2 input
function y = fcn(pos_1, pos_2)

y = cos(pos_1).*cos(pos_2);

== matlab function Simulation_1_3_dof/Signal 3 ==
  data: u input; y output; data_inYZ parameter; trial_length parameter
function y = fcn(u, data_inYZ, trial_length)

%u is the clock time input

%u is the clock time input
x = mod(u, (trial_length+3));


%check_data = 0:0.01:10;
check_data = data_inYZ;


y_temp = 0;

%temp assignment to check if the model works
y=y_temp;

[numRows,numCols] = size(check_data);
loop = 1;

%disp(class(round((x./(step/2)).*numCols)))

i=round((x./(trial_length)).*numCols);
if i == 0
    i = 1;
end
if i>numCols
    i = numCols;
end
y_temp = check_data(1,i);


if x>=trial_length
    y = 0;
else
    y = y_temp;

end

== matlab function Simulation_1_3_dof/Subsystem1/((m2.*(L2//2)^2)+(m3.*(L2^2))) ==
  data: signal_in input; y output; m3_state input; m3 parameter; m3_new parameter; L2 parameter; m2 parameter
function y  = fcn(signal_in,m3_state,m3, m3_new, L2, m2)

m3_temp = 0;
if m3_state == 1
    m3_temp = m3_new;
else
    m3_temp = m3;
end

y = signal_in .* ((m2.*(L2/2)^2)+(m3_temp.*(L2^2)));

== matlab function Simulation_1_3_dof/Subsystem1/1//( (m1.*(L1//2)^2)+(m2.*L1^2)+(m3.*L1^2)) ==
  data: signal_in input; y output; m3_state input; m3 parameter; m3_new parameter; L1 parameter; m2 parameter; m1 parameter
function y  = fcn(signal_in,m3_state,m3, m3_new, L1, m2, m1)

m3_temp = 0;

if m3_state == 1
    m3_temp = m3_new;
else
    m3_temp = m3;
end

y = signal_in .* (1/((m1.*(L1/2)^2)+(m2.*L1^2)+(m3_temp.*L1^2)));

== matlab function Simulation_1_3_dof/Subsystem1/1//( (m2.*(L2//2)^2)+(m3.*(L2^2))) ==
  data: signal_in input; y output; m3_state input; m3 parameter; m3_new parameter; L2 parameter; m2 parameter
function y  = fcn(signal_in,m3_state,m3, m3_new, L2, m2)

m3_temp = 0;

if m3_state == 1
    m3_temp = m3_new;
else
    m3_temp = m3;
end

y = signal_in .* (1/((m2.*(L2/2)^2)+(m3_temp.*(L2^2))));

== matlab function Simulation_1_3_dof/m3 signal ==
  data: u input; y output; trial_length parameter; m3_new parameter; m3_state_input parameter; m3 parameter
function y = fcn(u, trial_length, m3_new, m3_state_input, m3)

%u is the clock time input
x = mod(u, (trial_length+3));

%check_data = 0:0.01:10;
check_data = m3_state_input;
y_temp = 0;

[numRows,numCols] = size(check_data);

%disp(class(round((x./(step/2)).*numCols)))
i=round((x./(trial_length)).*numCols);
if i == 0
    i = 1;
end
if i>numCols
    i = numCols;
end
y_temp = check_data(1,i);



if x>=trial_length
    y = m3;
else
    if y_temp == 1
        y = m3_new;
    else 
        y = m3;
    end

end
